simulink model "Drone_Simulink_Model_SAAS_variable_trajectory"  (R2024b)
settings: Solver=ode45  StartTime=0.0  StopTime=800  RelTol=1e-9  EnableMultiTasking=on
StopFcn:
  | x = X;
  | r = ref;
  | plot3(x(:,1), x(:,3), x(:,5), 'r-', LineWidth=1.5);
  | grid on;
  | hold on;
  | plot3(r(:,1), r(:,2), r(:,3), 'k--', LineWidth=1.5);
  | hold off;
values from neighbouring files (symbols this model uses):
  K2 = acker(A2, B2, p)    [kval.m]
undefined symbols (not defined in the file or in its folder): K1
settings Model: Creator=Dalil  LastModifiedBy=user
settings SolverCC: AlgebraicLoopSolver=TrustRegion
settings DataIOCC: LimitDataPoints=on  SaveFormat=Array  ReturnWorkspaceOutputs=off
settings OptimizationCC: ExpressionDepthLimit=2147483647  LifeSpan=inf
settings DebuggingCC: UnderspecifiedInitializationDetection=Classic  MergeDetectMultiDrivingBlocksExec=none  SolverPrmCheckMsg=warning  UnconnectedInputMsg=warning  UnconnectedOutputMsg=warning  UnconnectedLineMsg=warning  StateNameClashWarn=warning  SFUnexpectedBacktrackingDiag=warning  SFNoUnconditionalDefaultTransitionDiag=warning  SFExecutionAtInitializationDiag=none  ArithmeticOperatorsInVariantConditions=warning
settings HardwareCC: ProdBitPerPointer=32  ProdBitPerSizeT=32  ProdBitPerPtrDiffT=32  ProdLargestAtomicFloat=None  ProdIntDivRoundTo=Undefined  ProdEndianess=Unspecified  ProdWordSize=32  ProdHWDeviceType=32-bit Generic
settings ModelReferenceCC: EnableRefExpFcnMdlSchedulingChecks=on  PropagateSignalLabelsOutOfModel=off
settings SFSimCC: SimUseLocalCustomCode=off  CustomCodeUndefinedFunction=UseInterfaceOnly
settings RTWCC: RTWUseLocalCustomCode=off  GPUComputeCapability=3.5  DLArmComputeVersion=19.05
settings CodeAppCC: StateflowObjectComments=on
settings GRTTargetCC: TargetLangStandard=C89/C90 (ANSI)
settings ConfigComp: CovMetricSettings=dw  CovSaveCumulativeToWorkspaceVar=on  CovSaveSingleToWorkspaceVar=on  CovExternalEMLEnable=off

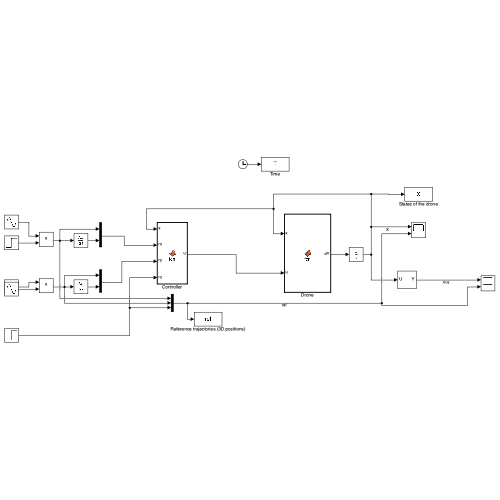
[thumbnail: Simulink's stored preview of the top-level diagram]
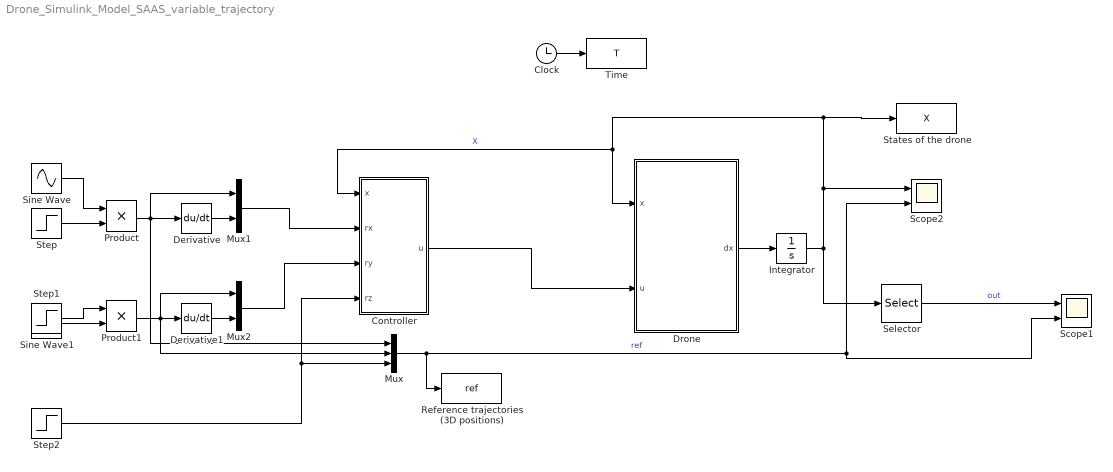
== system Drone_Simulink_Model_SAAS_variable_trajectory ==
  Clock : Clock
  Controller : MATLAB Function  TreatAsAtomicUnit=on
  Derivative : Derivative
  Derivative1 : Derivative
  Drone : MATLAB Function  TreatAsAtomicUnit=on
  Integrator : Integrator  InitialCondition=0.01*[1 1 1 1 1 1 1 1 1 1 1 1]
  Mux : Mux  Inputs=3
  Mux1 : Mux  Inputs=2
  Mux2 : Mux  Inputs=2
  Product : Product
  Product1 : Product
  Reference trajectories (3D positions) : ToWorkspace  VariableName=ref  SampleTime=-1
  Scope1 : Scope  NumInputPorts=2
  Scope2 : Scope  NumInputPorts=2
  Selector : Selector  InputPortWidth=12  IndexOptions=Index vector (dialog)  Indices=[1 3 5]  OutputSizes=1
  Sine Wave : Sin  Amplitude=2  Frequency=.01  SampleTime=0
  Sine Wave1 : Sin  Frequency=.01  Phase=pi/2  SampleTime=0
  States of the drone : ToWorkspace  VariableName=X  SampleTime=-1
  Step : Step  Time=10  SampleTime=0
  Step1 : Step  Time=20  SampleTime=0
  Step2 : Step  Time=0  SampleTime=0
  Time : ToWorkspace  VariableName=T  SampleTime=-1
  wires:
  Drone/1(dx) -> Integrator/1
  Integrator/1 -> Selector/1, Scope2/1, Drone/1(x), Controller/1(x), States of the drone/1  "X"
  Controller/1(u) -> Drone/2(u)
  Step2/1 -> Mux/3, Controller/4(rz)
  Mux/1 -> Reference trajectories (3D positions)/1, Scope1/2, Scope2/2  "ref"
  Clock/1 -> Time/1
  Step/1 -> Product/2
  Sine Wave/1 -> Product/1
  Product/1 -> Mux/1, Mux1/1, Derivative/1
  Product1/1 -> Mux/2, Derivative1/1, Mux2/1
  Step1/1 -> Product1/1
  Sine Wave1/1 -> Product1/2
  Selector/1 -> Scope1/1  "out"
  Derivative/1 -> Mux1/2
  Derivative1/1 -> Mux2/2
  Mux2/1 -> Controller/3(ry)
  Mux1/1 -> Controller/2(rx)

== matlab function Drone_Simulink_Model_SAAS_variable_trajectory/Controller ==
  data: x input; u output; rx input; ry input; rz input; K2 parameter; K1 parameter
function u = fcn(x,rx,ry,rz, K2, K1) % V_mat1, V_mat2,
%#codegen



u = zeros(6,1);

g  = 9.81;

% les moments inirtiels 
Ixx=7.5*10^-3;
Iyy=7.5*10^-3;
Izz=1.3*10^-3;

k1 = 2; k2 = 3;
k3 = 3; k4 = 5;
k5 = 9; k6 = 6;
k7 = 2; k8 = 3;
k9 = 2; k10 = 6;
k11 = 2; k12 = 3;

% les coeficients 
a1=((Iyy-Izz)/Ixx);
a2=((Izz-Ixx)/Iyy);
a3=((Ixx-Iyy)/Izz);

% % LQR + pole placement method
% % longitudinal
% xlong = [x(1); x(2); x(9); x(10)];
% u(1) = -K1*xlong+V_mat1(1)*rx(1); % To be completed;
% 
% % lateral 
% xlat = [x(3); x(4); x(7); x(8)];
% u(2) = -K2*xlat + V_mat2(1)*ry(1); % To be completed;


% u(3) = -(x(10)*x(2)-x(8)*x(4)+g*cos(x(7))*cos(x(9)))-k5*(x(5)-rz)-k6*x(6);
% u(4) = -(a1*x(12)*x(10))-k7*x(7)-k8*x(8);
% 

% exact linearization
% longitudinal control
u(1) = K1(1)*(rx(1)-x(1))+K1(2)*(rx(2)-x(2))-(x(12)*x(4)-x(10)*x(6)-g*sin(x(9)));

% lateral control

u(2) = K2(1)*(ry(1)-x(3))+K2(2)*(ry(2)-x(4))-(x(8)*x(6)-x(12)*x(2)+g*sin(x(7))*cos(x(9)));

u(3) = -k5*(x(5)-rz)-k6*x(6)-(x(10)*x(2)-x(4)*x(8)+g*cos(x(9))*cos(x(7)));
u(4) = -k7*x(11)-k8*x(12)-a3*x(10)*x(8);


u(5) = -a2*x(12)*x(8)-k9*x(9)-k10*x(10);
u(6) = -k11*x(7)-k12*x(8)-a1*x(12)*x(10);

== matlab function Drone_Simulink_Model_SAAS_variable_trajectory/Drone ==
  data: x input; u input; dx output
function dx = fcn(x,u)
%#codegen

g  = 9.81;

% les moments inirtiels 
Ixx=7.5*10^-3;
Iyy=7.5*10^-3;
Izz=1.3*10^-3;


% les coeficients 
a1=((Iyy-Izz)/Ixx);
a2=((Izz-Ixx)/Iyy);
a3=((Ixx-Iyy)/Izz);

dx = zeros(12,1);

dx(1) = x(2);
dx(2) = x(12)*x(4)-x(10)*x(6)-g*sin(x(9))+u(1);
dx(3) = x(4);
dx(4) = x(8)*x(6)-x(12)*x(2)+g*sin(x(7))*cos(x(9))+u(2);
dx(5) = x(6);
dx(6) = x(10)*x(2)-x(8)*x(4)+g*cos(x(7))*cos(x(9))+u(3);
dx(7) = x(8);
dx(8) = a1*x(12)*x(10)+u(6);
dx(9) = x(10);
dx(10) = a2*x(12)*x(8)+u(1);
dx(11) = x(12);
dx(12) = a3*x(8)*x(10)+u(4)+u(5);
